simulink model "brinsonSMA"  (R2020b)
settings: Solver=VariableStepAuto  StartTime=0.0  StopTime=10.0  RelTol=1e-3
settings Model: Creator=Jack  LastModifiedBy=Jack

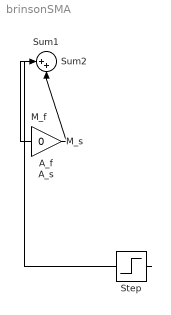
== system brinsonSMA ==
  A_f : Gain  Gain=0
  A_s : Gain  Gain=0
  M_f : Gain  Gain=0
  M_s : Gain  Gain=0
  Step : Step  Time=0  SampleTime=0
  Sum1 : Sum  Inputs=|++
  Sum2 : Sum  Inputs=|++
  wires:
  Step/1 -> Sum1/1
  A_s/1 -> Sum1/2
  A_f/1 -> Sum2/1
  M_s/1 -> Sum2/2
